simulink model "data_collection"  (R2024a)
settings: Solver=FixedStepAuto  StartTime=0.0  StopTime=inf  RelTol=1e-3
undefined symbols (not defined in the file or in its folder): X, Y, Z
libraries: robotlib x4, simulink x2, sharedtransform x1, simulink_extras x1
settings Model: Creator=hmcl  LastModifiedBy=hmcl
settings OptimizationCC: EnhancedBackFolding=on  PassReuseOutputArgsAs=Individual arguments  ZeroExternalMemoryAtStartup=off  ZeroInternalMemoryAtStartup=off  MaxStackSize=64  OptimizeBlockOrder=speed  DifferentSizesBufferReuse=on  OptimizationCustomize=off  EfficientTunableParamExpr=on
settings DebuggingCC: ParameterTunabilityLossMsg=error
settings HardwareCC: ProdBitPerPointer=32  ProdBitPerSizeT=32  ProdBitPerPtrDiffT=32  ProdLargestAtomicFloat=None  ProdIntDivRoundTo=Undefined  ProdEndianess=Unspecified  ProdWordSize=32  ProdHWDeviceType=Generic->Unspecified (assume 32-bit Generic)
settings SFSimCC: MATLABDynamicMemAlloc=off
settings RTWCC: Description=Embedded Coder  SystemTargetFile=ert.tlc  HardwareBoard=Robot Operating System (ROS)  TLCOptions="-aInlineSetEventsForThisBaseRateFcn=TLC_FALSE -aSuppressMultiTaskScheduler=TLC_FALSE  -aRateBasedStepFcn=0"  TemplateMakefile=ert_default_tmf  Toolchain=Catkin  TargetLang=C++  GPUComputeCapability=3.5
settings CodeAppCC: ForceParamTrailComments=on  IgnoreCustomStorageClasses=off  OperatorAnnotations=on  SimulinkDataObjDesc=on  SFDataObjDesc=on  InsertBlockDesc=on

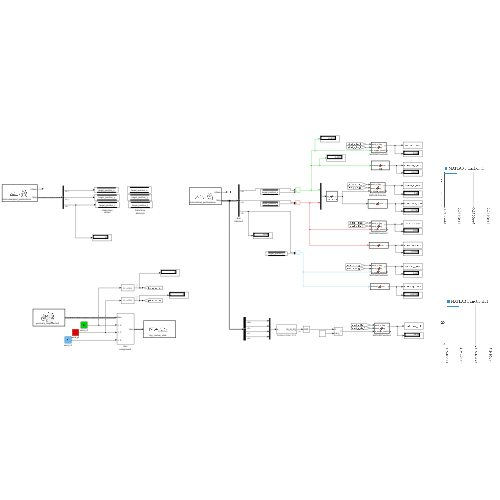
[thumbnail: Simulink's stored preview of the top-level diagram]
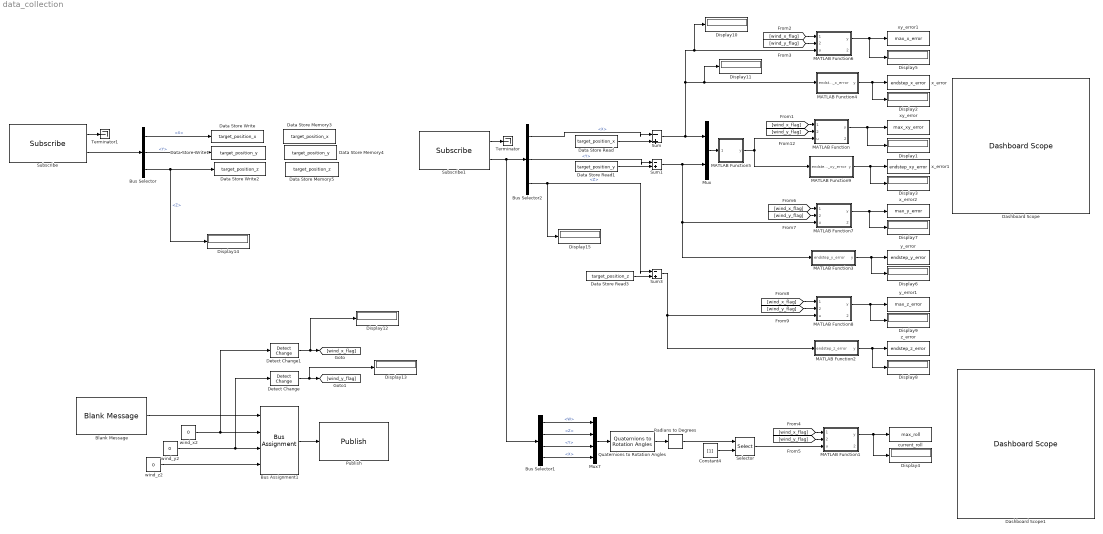
== system data_collection ==
  Blank Message : robotlib/Blank Message  messageClass=Message  entityType=geometry_msgs/Vector3  messageType=geometry_msgs/Vector3  SampleTime=inf  legacyBusStruct=off
  Bus Assignment1 : BusAssignment  AssignedSignals=X,Y,Z
  Bus Selector : BusSelector  OutputSignals=Pose.Position.X,Pose.Position.Y,Pose.Position.Z
  Bus Selector1 : BusSelector  OutputSignals=Pose.Orientation.W,Pose.Orientation.Z,Pose.Orientation.Y,Pose.Orientation.X
  Bus Selector2 : BusSelector  OutputSignals=Pose.Position.X,Pose.Position.Y,Pose.Position.Z
  Constant4 : Constant  Value=[1]
  Dashboard Scope : DashboardScope
  Dashboard Scope1 : DashboardScope
  Data Store Memory3 : DataStoreMemory  DataStoreName=target_position_x  ReadBeforeWriteMsg=warning  WriteAfterWriteMsg=warning  WriteAfterReadMsg=warning  ShowAdditionalParam=off
  Data Store Memory4 : DataStoreMemory  DataStoreName=target_position_y  ReadBeforeWriteMsg=warning  WriteAfterWriteMsg=warning  WriteAfterReadMsg=warning  ShowAdditionalParam=off
  Data Store Memory5 : DataStoreMemory  DataStoreName=target_position_z  ReadBeforeWriteMsg=warning  WriteAfterWriteMsg=warning  WriteAfterReadMsg=warning  ShowAdditionalParam=off
  Data Store Read : DataStoreRead  DataStoreName=target_position_x  IndexOptions=Index vector (dialog)  Indices=1  OutputSizes=1
  Data Store Read1 : DataStoreRead  DataStoreName=target_position_y  IndexOptions=Index vector (dialog)  Indices=1  OutputSizes=1
  Data Store Read3 : DataStoreRead  DataStoreName=target_position_z  IndexOptions=Index vector (dialog)  Indices=1  OutputSizes=1
  Data Store Write : DataStoreWrite  DataStoreName=target_position_x  IndexOptions=Index vector (dialog)  Indices=1  OutputSizes=1
  Data Store Write1 : DataStoreWrite  DataStoreName=target_position_y  IndexOptions=Index vector (dialog)  Indices=1  OutputSizes=1
  Data Store Write2 : DataStoreWrite  DataStoreName=target_position_z  IndexOptions=Index vector (dialog)  Indices=1  OutputSizes=1
  Detect Change : simulink/Logic and Bit Operations/Detect Change  vinit=0  OutDataTypeStr=boolean
  Detect Change1 : simulink/Logic and Bit Operations/Detect Change  vinit=0  OutDataTypeStr=boolean
  Display{1..15} (15 alike) : Display
  MATLAB Function : MATLAB Function  TreatAsAtomicUnit=on
  MATLAB Function1 : MATLAB Function  TreatAsAtomicUnit=on
  MATLAB Function2 : MATLAB Function  TreatAsAtomicUnit=on
  MATLAB Function3 : MATLAB Function  TreatAsAtomicUnit=on
  MATLAB Function4 : MATLAB Function  TreatAsAtomicUnit=on
  MATLAB Function5 : MATLAB Function  TreatAsAtomicUnit=on
  MATLAB Function6 : MATLAB Function  TreatAsAtomicUnit=on
  MATLAB Function7 : MATLAB Function  TreatAsAtomicUnit=on
  MATLAB Function8 : MATLAB Function  TreatAsAtomicUnit=on
  MATLAB Function9 : MATLAB Function  TreatAsAtomicUnit=on
  Mux : Mux  Inputs=2
  Mux7 : Mux
  Publish : robotlib/Publish  topicSource=Select from ROS network  topic=/my_custom_wind  messageType=geometry_msgs/Vector3  legacyBusStruct=off  messageQueueLength=1
  Quaternions to Rotation Angles : sharedtransform/Quaternions to Rotation Angles  rotationOrder=ZYX  aMode=aMode
  Radians to Degrees : simulink_extras/Transformations/Radians to Degrees
  Selector : Selector  InputPortWidth=3  IndexOptions=Index vector (port)  Indices=[1 3]  OutputSizes=1
  Subscribe : robotlib/Subscribe  topicSource=Select from ROS network  topic=/mavros/setpoint_position/local  messageType=geometry_msgs/PoseStamped  SampleTime=-1  legacyBusStruct=off  messageQueueLength=1
  Subscribe1 : robotlib/Subscribe  topicSource=Select from ROS network  topic=/mavros/local_position/pose  messageType=geometry_msgs/PoseStamped  SampleTime=-1  legacyBusStruct=off  messageQueueLength=1
  Sum : Sum  Inputs=|-+
  Sum1 : Sum  Inputs=|-+
  Sum3 : Sum  Inputs=|-+
  Terminator : Terminator
  Terminator1 : Terminator
  current_roll : ToWorkspace  VariableName=max_roll  SampleTime=-1
      settings: Save2DSignal=2-D array (concatenate along first dimension)
  wind_x2 : Constant  Value=0
  wind_y2 : Constant  Value=0
  wind_z2 : Constant  Value=0
  x_error : ToWorkspace  VariableName=endstep_x_error  SampleTime=-1
      settings: Save2DSignal=2-D array (concatenate along first dimension)
  x_error1 : ToWorkspace  VariableName=endstep_xy_error  SampleTime=-1
      settings: Save2DSignal=2-D array (concatenate along first dimension)
  x_error2 : ToWorkspace  VariableName=max_y_error  SampleTime=-1
      settings: Save2DSignal=2-D array (concatenate along first dimension)
  xy_error : ToWorkspace  VariableName=max_xy_error  SampleTime=-1
      settings: Save2DSignal=2-D array (concatenate along first dimension)
  xy_error1 : ToWorkspace  VariableName=max_x_error  SampleTime=-1
      settings: Save2DSignal=2-D array (concatenate along first dimension)
  y_error : ToWorkspace  VariableName=endstep_y_error  SampleTime=-1
      settings: Save2DSignal=2-D array (concatenate along first dimension)
  y_error1 : ToWorkspace  VariableName=max_z_error  SampleTime=-1
      settings: Save2DSignal=2-D array (concatenate along first dimension)
  z_error : ToWorkspace  VariableName=endstep_z_error  SampleTime=-1
      settings: Save2DSignal=2-D array (concatenate along first dimension)
  wires:
  Subscribe1/1 -> Terminator/1
  Bus Selector/3 -> Display14/1, Data Store Write2/1  "<Z>"
  Subscribe/1 -> Terminator1/1
  Bus Selector/2 -> Data Store Write1/1  "<Y>"
  Bus Selector/1 -> Data Store Write/1  "<X>"
  Detect Change1/1 -> Display12/1, [wind_x_flag]
  Detect Change/1 -> Display13/1, [wind_y_flag]
  Bus Assignment1/1 -> Publish/1
  Blank Message/1 -> Bus Assignment1/1
  wind_x2/1 -> Detect Change1/1, Bus Assignment1/2
  wind_y2/1 -> Detect Change/1, Bus Assignment1/3
  wind_z2/1 -> Bus Assignment1/4
  MATLAB Function3/1(y) -> Display6/1, y_error/1
  MATLAB Function2/1(y) -> Display8/1, z_error/1
  MATLAB Function6/1(y) -> Display5/1, xy_error1/1
  MATLAB Function7/1(y) -> Display7/1, x_error2/1
  MATLAB Function/1(y) -> Display1/1, xy_error/1
  MATLAB Function4/1(y) -> x_error/1, Display2/1
  MATLAB Function8/1(y) -> Display9/1, y_error1/1
  MATLAB Function9/1(y) -> x_error1/1, Display3/1
  Data Store Read/1 -> Sum/2
  [wind_x_flag] -> MATLAB Function6/1(wind_x_flag)
  [wind_x_flag] -> MATLAB Function7/1(wind_x_flag)
  Sum3/1 -> MATLAB Function2/1(endstep_z_error), MATLAB Function8/3(u)
  [wind_y_flag] -> MATLAB Function/2(wind_y_flag)
  Bus Selector2/2 -> Sum1/1  "<Y>"
  [wind_x_flag] -> MATLAB Function/1(wind_x_flag)
  MATLAB Function5/1(y) -> MATLAB Function9/1(endstep_xy_error), MATLAB Function/3(u)
  [wind_x_flag] -> MATLAB Function8/1(wind_x_flag)
  Data Store Read3/1 -> Sum3/2
  Bus Selector2/1 -> Sum/1  "<X>"
  Bus Selector2/3 -> Display15/1, Sum3/1  "<Z>"
  [wind_y_flag] -> MATLAB Function7/2(wind_y_flag)
  Mux/1 -> MATLAB Function5/1(xy_error)
  [wind_y_flag] -> MATLAB Function8/2(wind_y_flag)
  Sum/1 -> Display10/1, MATLAB Function6/3(u), Display11/1, MATLAB Function4/1(endstep_x_error), Mux/1
  Sum1/1 -> MATLAB Function7/3(u), MATLAB Function3/1(endstep_y_error), Mux/2
  Data Store Read1/1 -> Sum1/2
  [wind_y_flag] -> MATLAB Function6/2(wind_y_flag)
  MATLAB Function1/1(y) -> Display4/1, current_roll/1
  Constant4/1 -> Selector/2
  Quaternions to Rotation Angles/1 -> Radians to Degrees/1
  Bus Selector1/3 -> Mux7/3  "<Y>"
  Mux7/1 -> Quaternions to Rotation Angles/1
  Selector/1 -> MATLAB Function1/3(u)
  [wind_x_flag] -> MATLAB Function1/1(wind_x_flag)
  Bus Selector1/4 -> Mux7/4  "<X>"
  Bus Selector1/1 -> Mux7/1  "<W>"
  Bus Selector1/2 -> Mux7/2  "<Z>"
  [wind_y_flag] -> MATLAB Function1/2(wind_y_flag)
  Radians to Degrees/1 -> Selector/1
  Subscribe/2 -> Bus Selector/1
  Subscribe1/2 -> Bus Selector1/1, Bus Selector2/1

== matlab function data_collection/MATLAB Function1 ==
  data: wind_x_flag input; wind_y_flag input; u input; y output; toggle_swtich output
function [y, toggle_swtich] = fcn(wind_x_flag, wind_y_flag, u)
    coder.extrinsic('assignin'); % MATLAB 함수 사용을 알림


    % 이전 값을 저장할 persistent 변수 선언
    persistent prev_u;
    persistent toggle_state;

    if isempty(prev_u)
        prev_u = -inf; % 초기 값 설정
    end

    if isempty(toggle_state)
        toggle_state = false; % 초기 토글 상태를 논리형으로 설정
    end

    if wind_x_flag || wind_y_flag
        % 토글 상태를 변경
        toggle_state = ~toggle_state;      
    end

    % 현재 토글 상태를 int32 형으로 변환하여 할당
    toggle_swtich = int32(toggle_state);
    % 현재 토글 상태를 출력
    % fprintf('toggle_state = %d \n', toggle_swtich);

    if toggle_state
        % 현재 값이 이전 값보다 큰지 확인
        if abs(u) > abs(prev_u)
            
            prev_u = abs(u); % 이전 값을 현재 값으로 업데이트
            y = abs(u); % 현재 값을 출력
        else
            y = abs(prev_u); % 이전 값을 출력
        end
        assignin('base', 'max_roll', y); % y 값을 MATLAB 기본 워크스페이스의 current_roll에 저장
    else
        % 토글 상태가 0일 때
        prev_u = 0;
        y = 0;
    end
end




    % if x_change || y_change
    % 
    %     % 현재 값이 이전 값보다 큰지 확인
    %     if u > prev_u
    %         assignin('base', 'current_roll', u);  % u 값을 MATLAB  워크스페이스(base는 MATLAB의 기본 워크스페이스를 의미)의 current_roll에 저장
    %         prev_u = u; % 이전 값을 현재 값으로 업데이트
    %         y = u; % 현재 값을 출력
    %     else
    %         y = prev_u; % 이전 값을 출력
    %     end
    % else
    %     assignin('base', 'current_roll', u);
    %     y = 0;
    % end

== matlab function data_collection/MATLAB Function ==
  data: wind_x_flag input; wind_y_flag input; u input; y output; toggle_swtich output
function [y, toggle_swtich] = fcn(wind_x_flag, wind_y_flag, u)
    coder.extrinsic('assignin'); % MATLAB 함수 사용을 알림


    % 이전 값을 저장할 persistent 변수 선언
    persistent prev_u;
    persistent toggle_state;

    if isempty(prev_u)
        prev_u = -inf; % 초기 값 설정
    end

    if isempty(toggle_state)
        toggle_state = false; % 초기 토글 상태를 논리형으로 설정
    end

    if wind_x_flag || wind_y_flag
        % 토글 상태를 변경
        toggle_state = ~toggle_state;      
    end

    % 현재 토글 상태를 int32 형으로 변환하여 할당
    toggle_swtich = int32(toggle_state);
    % 현재 토글 상태를 출력
    % fprintf('toggle_state = %d \n', toggle_swtich);

    if toggle_state
        % 현재 값이 이전 값보다 큰지 확인
        if u > prev_u
            
            prev_u = u; % 이전 값을 현재 값으로 업데이트
            y = u; % 현재 값을 출력
        else
            y = prev_u; % 이전 값을 출력
        end
        assignin('base', 'max_xy_error', y); % y 값을 MATLAB 기본 워크스페이스의 xy_error에 저장
    else
        % 토글 상태가 0일 때
        prev_u = 0;
        y = 0;
    end
end




    % if x_change || y_change
    % 
    %     % 현재 값이 이전 값보다 큰지 확인
    %     if u > prev_u
    %         assignin('base', 'xy_error', u);  % u 값을 MATLAB  워크스페이스(base는 MATLAB의 기본 워크스페이스를 의미)의 xy_error에 저장
    %         prev_u = u; % 이전 값을 현재 값으로 업데이트
    %         y = u; % 현재 값을 출력
    %     else
    %         y = prev_u; % 이전 값을 출력
    %     end
    % else
    %     assignin('base', 'xy_error', u);
    %     y = 0;
    % end

== matlab function data_collection/MATLAB Function2 ==
  data: endstep_z_error input; y output
function y = fcn(endstep_z_error)

% z_error 값을 기본 워크스페이스에 저장
assignin('base', 'endstep_z_error', endstep_z_error);

% 저장된 값을 반환
y = endstep_z_error;

end

== matlab function data_collection/MATLAB Function3 ==
  data: endstep_y_error input; y output
function y = fcn(endstep_y_error)

% z_error 값을 기본 워크스페이스에 저장
assignin('base', 'endstep_y_error', endstep_y_error);

% 저장된 값을 반환
y = endstep_y_error;

end

== matlab function data_collection/MATLAB Function4 ==
  data: endstep_x_error input; y output
function y = fcn(endstep_x_error)

% z_error 값을 기본 워크스페이스에 저장
assignin('base', 'endstep_x_error', endstep_x_error);

% 저장된 값을 반환
y = endstep_x_error;

end

== matlab function data_collection/MATLAB Function5 ==
  data: xy_error input; y output
function y = two_norm(xy_error)
    coder.extrinsic('norm'); % MATLAB 함수 사용을 알림
    
    

    
    % 'y'를 명확히 초기화
    y = 0; 
    
y = norm(xy_error,2);

== matlab function data_collection/MATLAB Function6 ==
  data: wind_x_flag input; wind_y_flag input; u input; y output; toggle_swtich output
function [y, toggle_swtich] = fcn(wind_x_flag, wind_y_flag, u)
    coder.extrinsic('assignin'); % MATLAB 함수 사용을 알림


    % 이전 값을 저장할 persistent 변수 선언
    persistent prev_u;
    persistent toggle_state;

    if isempty(prev_u)
        prev_u = -inf; % 초기 값 설정
    end

    if isempty(toggle_state)
        toggle_state = false; % 초기 토글 상태를 논리형으로 설정
    end

    if wind_x_flag || wind_y_flag
        % 토글 상태를 변경
        toggle_state = ~toggle_state;      
    end

    % 현재 토글 상태를 int32 형으로 변환하여 할당
    toggle_swtich = int32(toggle_state);
    % 현재 토글 상태를 출력
    % fprintf('toggle_state = %d \n', toggle_swtich);

    if toggle_state
        % 현재 값이 이전 값보다 큰지 확인
        if abs(u) > abs(prev_u)
            
            prev_u = abs(u); % 이전 값을 현재 값으로 업데이트
            y = abs(u); % 현재 값을 출력
        else
            y = abs(prev_u); % 이전 값을 출력
        end
        assignin('base', 'max_x_error', y); % y 값을 MATLAB 기본 워크스페이스의 current_roll에 저장
    else
        % 토글 상태가 0일 때
        prev_u = 0;
        y = 0;
    end
end




    % if x_change || y_change
    % 
    %     % 현재 값이 이전 값보다 큰지 확인
    %     if u > prev_u
    %         assignin('base', 'current_roll', u);  % u 값을 MATLAB  워크스페이스(base는 MATLAB의 기본 워크스페이스를 의미)의 current_roll에 저장
    %         prev_u = u; % 이전 값을 현재 값으로 업데이트
    %         y = u; % 현재 값을 출력
    %     else
    %         y = prev_u; % 이전 값을 출력
    %     end
    % else
    %     assignin('base', 'current_roll', u);
    %     y = 0;
    % end

== matlab function data_collection/MATLAB Function7 ==
  data: wind_x_flag input; wind_y_flag input; u input; y output; toggle_swtich output
function [y, toggle_swtich] = fcn(wind_x_flag, wind_y_flag, u)
    coder.extrinsic('assignin'); % MATLAB 함수 사용을 알림


    % 이전 값을 저장할 persistent 변수 선언
    persistent prev_u;
    persistent toggle_state;

    if isempty(prev_u)
        prev_u = -inf; % 초기 값 설정
    end

    if isempty(toggle_state)
        toggle_state = false; % 초기 토글 상태를 논리형으로 설정
    end

    if wind_x_flag || wind_y_flag
        % 토글 상태를 변경
        toggle_state = ~toggle_state;      
    end

    % 현재 토글 상태를 int32 형으로 변환하여 할당
    toggle_swtich = int32(toggle_state);
    % 현재 토글 상태를 출력
    % fprintf('toggle_state = %d \n', toggle_swtich);

    if toggle_state
        % 현재 값이 이전 값보다 큰지 확인
        if abs(u) > abs(prev_u)
            
            prev_u = abs(u); % 이전 값을 현재 값으로 업데이트
            y = abs(u); % 현재 값을 출력
        else
            y = abs(prev_u); % 이전 값을 출력
        end
        assignin('base', 'max_y_error', y); % y 값을 MATLAB 기본 워크스페이스의 current_roll에 저장
    else
        % 토글 상태가 0일 때
        prev_u = 0;
        y = 0;
    end
end




    % if x_change || y_change
    % 
    %     % 현재 값이 이전 값보다 큰지 확인
    %     if u > prev_u
    %         assignin('base', 'current_roll', u);  % u 값을 MATLAB  워크스페이스(base는 MATLAB의 기본 워크스페이스를 의미)의 current_roll에 저장
    %         prev_u = u; % 이전 값을 현재 값으로 업데이트
    %         y = u; % 현재 값을 출력
    %     else
    %         y = prev_u; % 이전 값을 출력
    %     end
    % else
    %     assignin('base', 'current_roll', u);
    %     y = 0;
    % end

== matlab function data_collection/MATLAB Function8 ==
  data: wind_x_flag input; wind_y_flag input; u input; y output; toggle_swtich output
function [y, toggle_swtich] = fcn(wind_x_flag, wind_y_flag, u)
    coder.extrinsic('assignin'); % MATLAB 함수 사용을 알림


    % 이전 값을 저장할 persistent 변수 선언
    persistent prev_u;
    persistent toggle_state;

    if isempty(prev_u)
        prev_u = -inf; % 초기 값 설정
    end

    if isempty(toggle_state)
        toggle_state = false; % 초기 토글 상태를 논리형으로 설정
    end

    if wind_x_flag || wind_y_flag
        % 토글 상태를 변경
        toggle_state = ~toggle_state;      
    end

    % 현재 토글 상태를 int32 형으로 변환하여 할당
    toggle_swtich = int32(toggle_state);
    % 현재 토글 상태를 출력
    % fprintf('toggle_state = %d \n', toggle_swtich);

    if toggle_state
        % 현재 값이 이전 값보다 큰지 확인
        if abs(u) > abs(prev_u)
            
            prev_u = abs(u); % 이전 값을 현재 값으로 업데이트
            y = abs(u); % 현재 값을 출력
        else
            y = abs(prev_u); % 이전 값을 출력
        end
        assignin('base', 'max_z_error', y); % y 값을 MATLAB 기본 워크스페이스의 current_roll에 저장
    else
        % 토글 상태가 0일 때
        prev_u = 0;
        y = 0;
    end
end




    % if x_change || y_change
    % 
    %     % 현재 값이 이전 값보다 큰지 확인
    %     if u > prev_u
    %         assignin('base', 'current_roll', u);  % u 값을 MATLAB  워크스페이스(base는 MATLAB의 기본 워크스페이스를 의미)의 current_roll에 저장
    %         prev_u = u; % 이전 값을 현재 값으로 업데이트
    %         y = u; % 현재 값을 출력
    %     else
    %         y = prev_u; % 이전 값을 출력
    %     end
    % else
    %     assignin('base', 'current_roll', u);
    %     y = 0;
    % end

== matlab function data_collection/MATLAB Function9 ==
  data: endstep_xy_error input; y output
function y = fcn(endstep_xy_error)

% z_error 값을 기본 워크스페이스에 저장
assignin('base', 'endstep_xy_error', endstep_xy_error);

% 저장된 값을 반환
y = endstep_xy_error;

end
